simulink model "wesrf_imc_model"  (R2020b)
settings: Solver=FixedStepDiscrete  StartTime=0.0  StopTime=inf  FixedStep=0.001  RelTol=1e-3  EnableMultiTasking=on
PreLoadFcn:
  | demos_common_configs();
undefined symbols (not defined in the file or in its folder): a, b, c, d, DiscIntNeverNeededParam, heave_a, heave_b, heave_c, heave_d
libraries: franka_simulink_library x5, simulink x3, franka_simulink_library_misc x2
settings Model: SimulationMode=external  ExtModeTrigDuration=30000  ExtModeArchiveMode=auto  ExtModeArchiveFileName=data  ExtModeArchiveDirName=/home/host/franka_matlab_v0.2.0/WESRF_workingDir/data/output_data  ExtModeAddSuffixToVar=on  ExtModeLogAll=off  Creator=vasi_ko  LastModifiedBy=root
settings DataIOCC: LimitDataPoints=on  SaveFormat=Array  ReturnWorkspaceOutputs=off
settings OptimizationCC: DefaultParameterBehavior=Inlined  EnhancedBackFolding=on  PassReuseOutputArgsAs=Individual arguments  ZeroExternalMemoryAtStartup=off  ZeroInternalMemoryAtStartup=off  OptimizeBlockOrder=speed  DifferentSizesBufferReuse=on  OptimizationCustomize=off  EfficientTunableParamExpr=on
settings DebuggingCC: SolverPrmCheckMsg=warning  ParameterTunabilityLossMsg=error  SFUnexpectedBacktrackingDiag=warning  SFNoUnconditionalDefaultTransitionDiag=warning  SFExecutionAtInitializationDiag=none  ArithmeticOperatorsInVariantConditions=warning
settings HardwareCC: ProdBitPerLong=64  ProdHWDeviceType=Intel->x86-64 (Linux 64)  TargetBitPerLong=64  TargetBitPerPointer=64  TargetBitPerSizeT=64  TargetBitPerPtrDiffT=64  TargetLongLongMode=on  TargetIntDivRoundTo=Zero  TargetEndianess=LittleEndian  TargetWordSize=64  TargetHWDeviceType=MATLAB Host
settings ModelReferenceCC: PropagateSignalLabelsOutOfModel=off
settings SFSimCC: SimUseLocalCustomCode=off  MATLABDynamicMemAlloc=off  CustomCodeUndefinedFunction=UseInterfaceOnly  SimTargetLang=C++
settings RTWCC: Description=Embedded Coder  SystemTargetFile=franka_emika_panda.tlc  GenCodeOnly=on  TemplateMakefile=ert_default_tmf  RTWVerbose=off  RTWUseLocalCustomCode=off  Toolchain=Franka Simulink | gmake (64-bit linux)  BuildConfiguration=Faster Runs  IncludeHyperlinkInReport=on  TargetLang=C++
settings CodeAppCC: ForceParamTrailComments=on  IgnoreCustomStorageClasses=off  OperatorAnnotations=on  SimulinkDataObjDesc=on  SFDataObjDesc=on  InsertBlockDesc=on
settings STFCustomTargetCC: TargetLangStandard=C99 (ISO)  MultiwordLength=256  GenerateSampleERTMain=on  ModelReferenceCompliant=off  ConcurrentExecutionCompliant=off  CombineOutputUpdateFcns=on  ERTCustomFileBanners=on  SupportNonInlinedSFcns=off  RemoveResetFunc=on  MATLABClassNameForMDSCustomization=Simulink.SoftwareTarget.ERTCustomization  GRTInterface=off  UseToolchainInfoCompliant=on  SystemTargetFile=franka_emika_panda.tlc
settings ERTTargetCC: TargetLangStandard=C99 (ISO)  GenerateSampleERTMain=on  ModelReferenceCompliant=off  ParMdlRefBuildCompliant=off  CompOptLevelCompliant=off  ConcurrentExecutionCompliant=off  SupportContinuousTime=on  ModelStepFunctionPrototypeControlCompliant=off  ExtMode=on  ExtModeMexArgs='172.16.0.1' 0 17725  InlinedParameterPlacement=NonHierarchical  ERTCustomFileTemplate=franka_emika_panda_file_process.tlc
settings ConfigComp: CovMetricSettings=dw  CovSaveCumulativeToWorkspaceVar=on  CovSaveSingleToWorkspaceVar=on  CovExternalEMLEnable=off  CovSFcnEnable=off

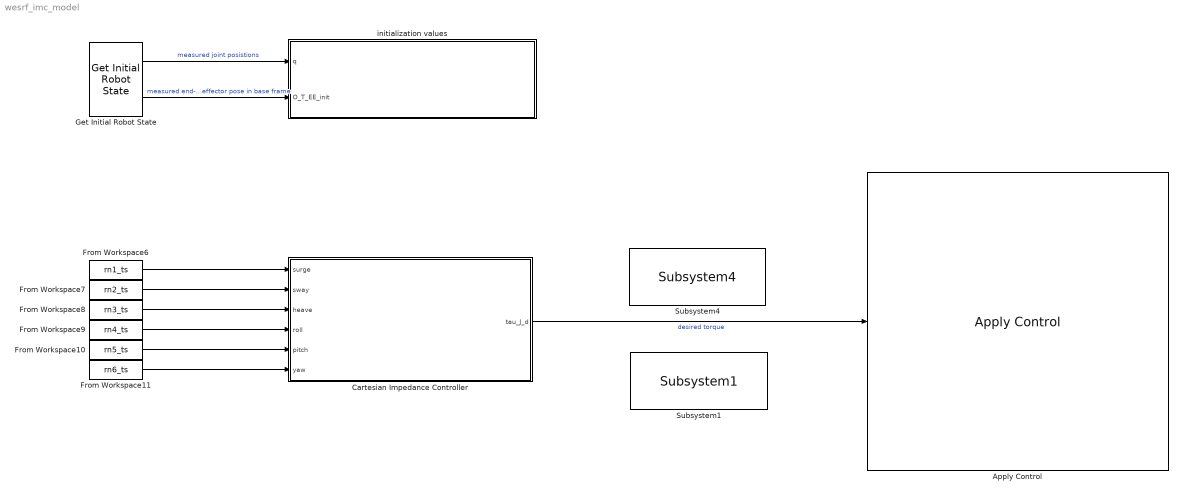
== system wesrf_imc_model ==
  Apply Control : franka_simulink_library/Apply Control  robot_ip=robot_ip  gripper_attached=off  control_mode=Torque Control  controller_choice=Joint Impedance Controller  elbow_control=on  collision_thresholds=100*ones(1,52)  joint_impedance=joint_impedance  cartesian_impedance=cartesian_impedance  load_inertia=load_inertia  EE_T_K=EE_T_K  init_joint_configuration_req=off  init_joint_configuration=[0.00392584915725334;-0.104076810189763;0.0404703493577216;-2.7334242600631;0.0113035300040543;2.63364770337236;0.372162046953987]
      settings: SourceProductName=Franka Emika
  Cartesian Impedance Controller : Subsystem
      mask Display:
      | disp('{\bf\fontsize{18}Force Controller}', 'texmode','on');
      | %
      | % block_icon('Controller')
      | %
      | port_label('input',1,'desired_mass');
      | port_label('output',1,'tau_J_d');
  From Workspace10 : FromWorkspace  VariableName=rn5_ts
  From Workspace11 : FromWorkspace  VariableName=rn6_ts
  From Workspace6 : FromWorkspace  VariableName=rn1_ts
  From Workspace7 : FromWorkspace  VariableName=rn2_ts
  From Workspace8 : FromWorkspace  VariableName=rn3_ts
  From Workspace9 : FromWorkspace  VariableName=rn4_ts
  Get Initial Robot State : franka_simulink_library/Get Initial Robot State  robot_ip=robot_ip  signals_requested='q O_T_EE'
      settings: SourceProductName=Franka Emika
  Subsystem1 : franka_simulink_library_misc/Subsystem1  SystemSampleTime=-1  VariantActivationTime=update diagram  Latency=0  AutoFrameSizeCalculation=off
  Subsystem4 : franka_simulink_library_misc/Subsystem4  SystemSampleTime=-1  VariantActivationTime=update diagram  Latency=0  AutoFrameSizeCalculation=off
  initialization values : Subsystem
  wires:
  Cartesian Impedance Controller/1(tau_J_d) -> Apply Control/1  "desired torque"
  Get Initial Robot State/1 -> initialization values/1(q)  "measured joint posistions"
  Get Initial Robot State/2 -> initialization values/2(O_T_EE_init)  "measured end-effector pose in base frame"
  From Workspace11/1 -> Cartesian Impedance Controller/6(yaw)
  From Workspace10/1 -> Cartesian Impedance Controller/5(pitch)
  From Workspace9/1 -> Cartesian Impedance Controller/4(roll)
  From Workspace8/1 -> Cartesian Impedance Controller/3(heave)
  From Workspace7/1 -> Cartesian Impedance Controller/2(sway)
  From Workspace6/1 -> Cartesian Impedance Controller/1(surge)

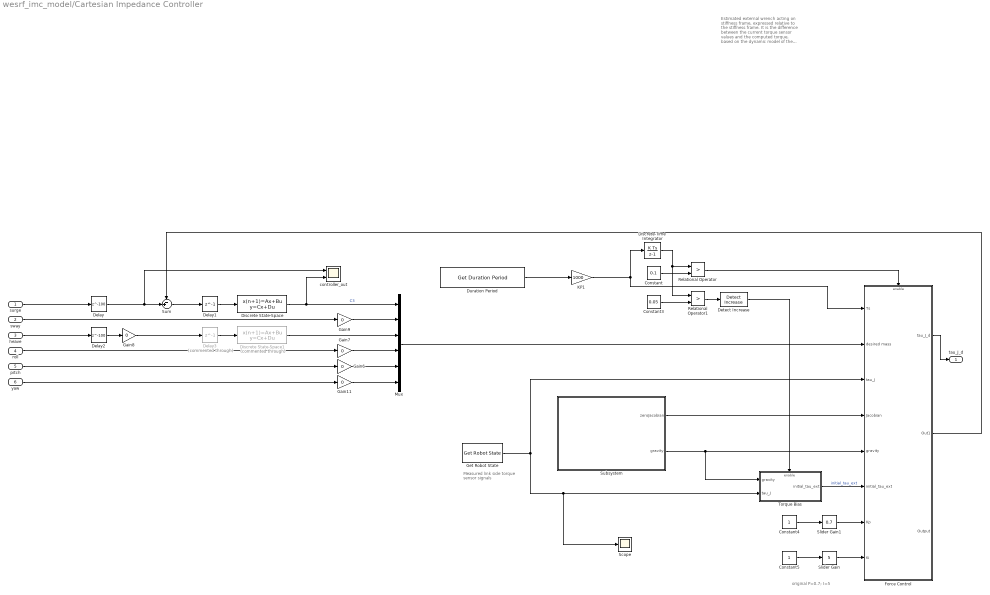
== system wesrf_imc_model/Cartesian Impedance Controller ==
  note: original P=0.7; I=5
  note: Measured link side torque sensor signals
  note: Estimated external wrench acting on stiffness frame, expressed relative to the stiffness frame. It is the difference between the current torque sensor values and the computed torque, based on the dynamic model of the robot.
  surge : Inport
  sway : Inport  Port=2
  heave : Inport  Port=3
  roll : Inport  Port=4
  pitch : Inport  Port=5
  yaw : Inport  Port=6
  Constant : Constant  Value=0.1
  Constant3 : Constant  Value=0.05
  Constant4 : Constant
  Constant5 : Constant
  Delay : Delay  DelayLength=100
  Delay1 : Delay  DelayLength=1
  Delay2 : Delay  DelayLength=100
  Delay3 : Delay  Commented=through  DelayLength=1
  Detect Increase : simulink/Logic and Bit Operations/Detect Increase  vinit=0.0  OutDataTypeStr=boolean
  Discrete State-Space : DiscreteStateSpace  A=a  B=b  C=c  D=d  SampleTime=1e-3
  Discrete State-Space1 : DiscreteStateSpace  Commented=through  A=heave_a  B=heave_b  C=heave_c  D=heave_d  SampleTime=1e-3
  Discrete-Time Integrator : DiscreteIntegrator  SampleTime=-1  ICPrevOutput=DiscIntNeverNeededParam  ICPrevScaledInput=DiscIntNeverNeededParam
  Duration Period : franka_simulink_library/Get Duration Period  robot_ip=robot_ip
      settings: SourceProductName=Franka Emika
  Force Control : Subsystem
  Gain{6..9,11} (5 alike) : Gain  Gain=0
  Get Robot State : franka_simulink_library/Get Robot State  robot_ip=robot_ip  signals_requested='tau_J'
      settings: SourceProductName=Franka Emika
  KP1 : Gain  Gain=1000
  Mux : Mux  Inputs=6
  Relational Operator : RelationalOperator  Operator=>  OutDataTypeStr=boolean  RndMeth=Nearest
  Relational Operator1 : RelationalOperator  Operator=>  OutDataTypeStr=boolean  RndMeth=Nearest
  Scope : Scope
  Slider Gain : simulink/Math Operations/Slider Gain  gain=5  low=1  high=12
  Slider Gain1 : simulink/Math Operations/Slider Gain  gain=0.7  low=0  high=2
  Subsystem : Subsystem
  Sum : Sum  Inputs=-+|
  Torque Bias : Subsystem
  controller_out : Scope  NumInputPorts=2
  tau_J_d : Outport  VectorParamsAs1DForOutWhenUnconnected=off
  wires:
  Get Robot State/1 -> Force Control/3(tau_J), Scope/1, Torque Bias/2(tau_J)
  Discrete-Time Integrator/1 -> Relational Operator1/1, Relational Operator/1
  Constant/1 -> Relational Operator/2
  KP1/1 -> Force Control/1(Ts), Discrete-Time Integrator/1
  Force Control/1(tau_J_d) -> tau_J_d/1
  Relational Operator/1 -> Force Control/Enable
  Duration Period/1 -> KP1/1
  Constant3/1 -> Relational Operator1/2
  Relational Operator1/1 -> Detect Increase/1
  Detect Increase/1 -> Torque Bias/Enable
  Subsystem/2(gravity) -> Torque Bias/1(gravity), Force Control/5(gravity)
  Subsystem/1(zeroJacobian) -> Force Control/4(Jacobian)
  Torque Bias/1(initial_tau_ext) -> Force Control/6(initial_tau_ext)  "initial_tau_ext"
  Constant5/1 -> Slider Gain/1
  Slider Gain/1 -> Force Control/8(Ki)
  Constant4/1 -> Slider Gain1/1
  Slider Gain1/1 -> Force Control/7(Kp)
  Mux/1 -> Force Control/2(desired mass)
  Gain6/1 -> Mux/5
  Gain7/1 -> Mux/4
  Gain9/1 -> Mux/2
  Gain11/1 -> Mux/6
  Discrete State-Space/1 -> controller_out/2, Mux/1  "C3"
  Sum/1 -> Delay1/1
  surge/1 -> Delay/1
  yaw/1 -> Gain11/1
  pitch/1 -> Gain6/1
  roll/1 -> Gain7/1
  heave/1 -> Delay2/1
  sway/1 -> Gain9/1
  Force Control/2(Out1) -> Sum/1
  Delay/1 -> controller_out/1, Sum/2
  Delay1/1 -> Discrete State-Space/1
  Delay2/1 -> Gain8/1
  Delay3/1 -> Discrete State-Space1/1
  Gain8/1 -> Delay3/1
  Discrete State-Space1/1 -> Mux/3

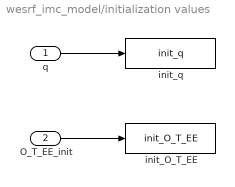
== system wesrf_imc_model/initialization values ==
  q : Inport
  O_T_EE_init : Inport  Port=2
  init_O_T_EE : ToWorkspace  VariableName=init_O_T_EE  SaveFormat=Structure With Time  SampleTime=-1
  init_q : ToWorkspace  VariableName=init_q  SaveFormat=Structure With Time  SampleTime=-1
  wires:
  q/1 -> init_q/1
  O_T_EE_init/1 -> init_O_T_EE/1

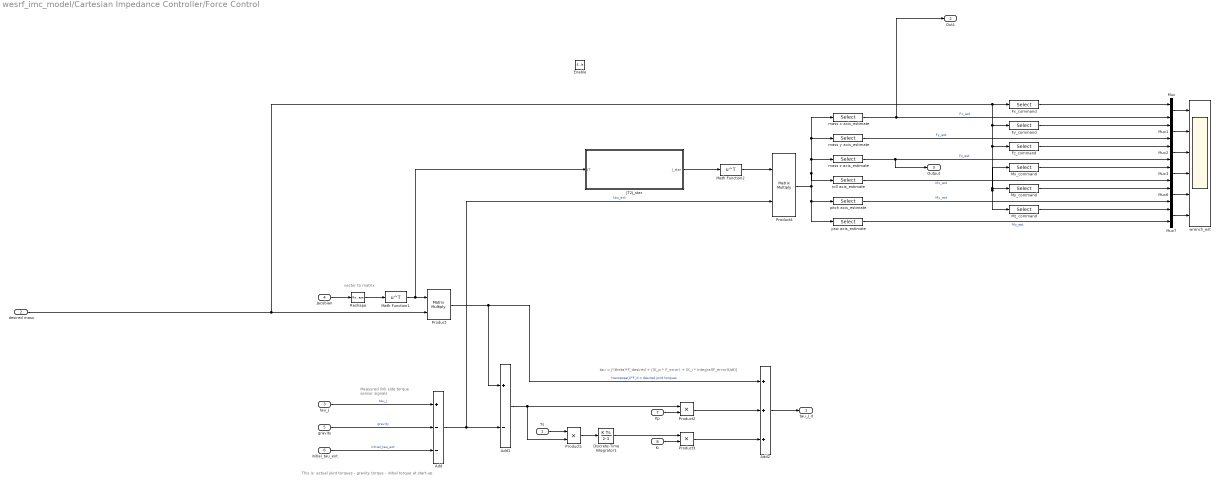
== system wesrf_imc_model/Cartesian Impedance Controller/Force Control ==
  note: This is: actual joint torques - gravity torque - initial torque at start-up
  note: vector to matrix
  note: tau = J'(theta)*F_desired + [(K_p * F_error) + (K_i * integral(F_error(t)dt)]
  note: Measured link side torque sensor signals
  Ts : Inport
  desired mass : Inport  Port=2
  tau_J : Inport  Port=3
  Jacobian : Inport  Port=4
  gravity : Inport  Port=5
  initial_tau_ext : Inport  Port=6
  Kp : Inport  Port=7
  Ki : Inport  Port=8
  Enable : EnablePort
  " roll axis_estimate" : Selector  InputPortWidth=6  IndexOptions=Index vector (dialog)  Indices=4  OutputSizes=1
  Add : Sum  Inputs=+--
  Add1 : Sum  Inputs=+-
  Add2 : Sum  Inputs=+++
  Discrete-Time Integrator1 : DiscreteIntegrator  SampleTime=0.001  ICPrevOutput=DiscIntNeverNeededParam  ICPrevScaledInput=DiscIntNeverNeededParam
  Fx_command : Selector  InputPortWidth=6  IndexOptions=Index vector (dialog)  Indices=1  OutputSizes=1
  Fy_command : Selector  InputPortWidth=6  IndexOptions=Index vector (dialog)  Indices=2  OutputSizes=1
  Fz_command : Selector  InputPortWidth=6  IndexOptions=Index vector (dialog)  Indices=3  OutputSizes=1
  JT2J_star : MATLAB Function  TreatAsAtomicUnit=on
  Math Function1 : Math  Operator=transpose  SignedPower=on  SaturateOnIntegerOverflow=on
  Math Function2 : Math  Operator=transpose  SignedPower=on  SaturateOnIntegerOverflow=on
  Mux{,1..3,6..7} (6 alike) : Mux  Inputs=2
  Mx_command : Selector  InputPortWidth=6  IndexOptions=Index vector (dialog)  Indices=4  OutputSizes=1
  My_command : Selector  InputPortWidth=6  IndexOptions=Index vector (dialog)  Indices=5  OutputSizes=1
  Mz_command : Selector  InputPortWidth=6  IndexOptions=Index vector (dialog)  Indices=6  OutputSizes=1
  Product : Product  Multiplication=Matrix(*)
  Product1 : Product
  Product2 : Product
  Product3 : Product
  Product4 : Product  Multiplication=Matrix(*)
  Reshape : Reshape  OutputDimensionality=Customize  OutputDimensions=[6,7]
  mass x axis_estimate : Selector  InputPortWidth=6  IndexOptions=Index vector (dialog)  Indices=1  OutputSizes=1
  mass y axis_estimate : Selector  InputPortWidth=6  IndexOptions=Index vector (dialog)  Indices=2  OutputSizes=1
  mass z axis_estimate : Selector  InputPortWidth=6  IndexOptions=Index vector (dialog)  Indices=3  OutputSizes=1
  pitch axis_estimate : Selector  InputPortWidth=6  IndexOptions=Index vector (dialog)  Indices=5  OutputSizes=1
  wrench_est : Scope  NumInputPorts=6
  yaw axis_estimate : Selector  InputPortWidth=6  IndexOptions=Index vector (dialog)  Indices=6  OutputSizes=1
  tau_J_d : Outport  InitialOutput=[0 0 0 0 0 0 0]  VectorParamsAs1DForOutWhenUnconnected=off
  Out1 : Outport  Port=2
  Output : Outport  Port=3
  wires:
  tau_J/1 -> Add/1  "tau_J"
  gravity/1 -> Add/2  "gravity"
  Add/1 -> Product4/2, Add1/2  "tau_ext"
  Add1/1 -> Product2/1, Product1/2
  Add2/1 -> tau_J_d/1
  Product1/1 -> Discrete-Time Integrator1/1
  Ts/1 -> Product1/1
  Product3/1 -> Add2/3
  initial_tau_ext/1 -> Add/3  "initial_tau_ext"
  Product/1 -> Add1/1, Add2/1  "transpose(J)*F_d = desired joint torques"
  Product2/1 -> Add2/2
  Discrete-Time Integrator1/1 -> Product3/1
  Jacobian/1 -> Reshape/1
  Reshape/1 -> Math Function1/1
  Kp/1 -> Product2/2
  Ki/1 -> Product3/2
  Math Function2/1 -> Product4/1
  JT2J_star/1(J_star) -> Math Function2/1
  Product4/1 -> " roll axis_estimate"/1, mass x axis_estimate/1, mass y axis_estimate/1, mass z axis_estimate/1, yaw axis_estimate/1, pitch axis_estimate/1
  Math Function1/1 -> JT2J_star/1(JT), Product/1
  Mux/1 -> wrench_est/1
  Fx_command/1 -> Mux/1
  Mux7/1 -> wrench_est/6
  Mux6/1 -> wrench_est/5
  Mux3/1 -> wrench_est/4
  Mux1/1 -> wrench_est/2
  Fy_command/1 -> Mux1/1
  Fz_command/1 -> Mux2/1
  Mx_command/1 -> Mux3/1
  My_command/1 -> Mux6/1
  Mz_command/1 -> Mux7/1
  mass x axis_estimate/1 -> Out1/1, Mux/2  "Fx_est"
  mass y axis_estimate/1 -> Mux1/2  "Fy_est"
  mass z axis_estimate/1 -> Output/1, Mux2/2  "Fz_est"
  " roll axis_estimate"/1 -> Mux3/2  "Mx_est"
  pitch axis_estimate/1 -> Mux6/2  "My_est"
  yaw axis_estimate/1 -> Mux7/2  "Mz_est"
  Mux2/1 -> wrench_est/3
  desired mass/1 -> Product/2, Mx_command/1, My_command/1, Mz_command/1, Fz_command/1, Fy_command/1, Fx_command/1

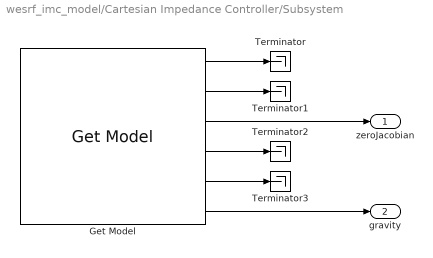
== system wesrf_imc_model/Cartesian Impedance Controller/Subsystem ==
  Get Model : franka_simulink_library/Get Model  robot_ip=robot_ip
      settings: SourceProductName=Franka Emika
  Terminator{,1..3} (4 alike) : Terminator
  zeroJacobian : Outport  VectorParamsAs1DForOutWhenUnconnected=off
  gravity : Outport  Port=2  VectorParamsAs1DForOutWhenUnconnected=off
  wires:
  Get Model/6 -> gravity/1
  Get Model/3 -> zeroJacobian/1
  Get Model/2 -> Terminator1/1
  Get Model/1 -> Terminator/1
  Get Model/5 -> Terminator3/1
  Get Model/4 -> Terminator2/1

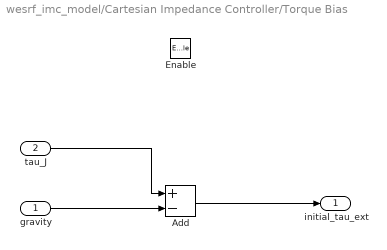
== system wesrf_imc_model/Cartesian Impedance Controller/Torque Bias ==
  gravity : Inport
  tau_J : Inport  Port=2
  Enable : EnablePort
  Add : Sum  Inputs=+-
  initial_tau_ext : Outport  InitialOutput=[0 0 0 0 0 0 0]  VectorParamsAs1DForOutWhenUnconnected=off
  wires:
  tau_J/1 -> Add/1
  gravity/1 -> Add/2
  Add/1 -> initial_tau_ext/1

== matlab function wesrf_imc_model/Cartesian Impedance Controller/Force Control/JT2J_star ==
  data: JT input; J_star output
function J_star = JT2J_star(JT)
%#codegen

J = JT';
% low isotropic damping, the value should be much smaller than lambda_max^2
beta =0;
% damping added in singular directions, we chose it to be equal to
% threshold
% lambda_max = singularity_threshold_inverse_kinematics; 
% SVD decomposition
[U,S,~] = svd(J);
sigma = diag(S);
% rank
singularity_threshold_inverse_kinematics = eps;
r = sum(sigma > singularity_threshold_inverse_kinematics);
% initilizing damping
  lambda_square_vector = zeros(6,1);
if r==6 % damping in full rank case is zero
    lambda_square_vector = zeros(6,1);
else % daamping in rank deficient cases
%     sigma_singular = sigma(r+1:6);
%     lambda_square_vector(r+1:6) = ...
%         (1 - (sigma_singular/ singularity_threshold_inverse_kinematics).^2) *...
%         lambda_max^2;
end
J_star =  JT * U * diag(1./(sigma.^2+lambda_square_vector+beta^2*ones(6,1)))*U';

end
